simulink model "task11"  (R2023a)
settings: Solver=ode15s  StartTime=0.0  StopTime=10.0  RelTol=1e-3
undefined symbols (not defined in the file or in its folder): DisplayTrajectoryImpedance
settings Model: Creator=LENOVO  LastModifiedBy=LENOVO

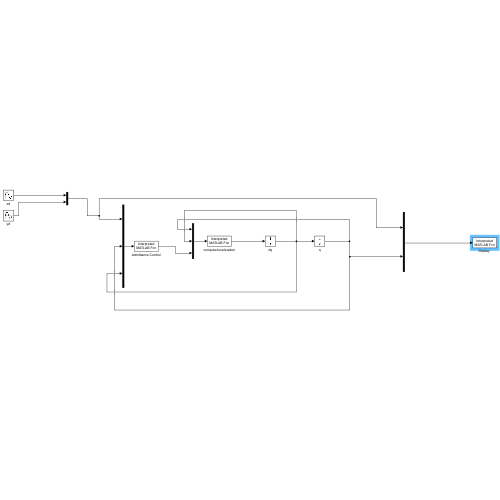
[thumbnail: Simulink's stored preview of the top-level diagram]
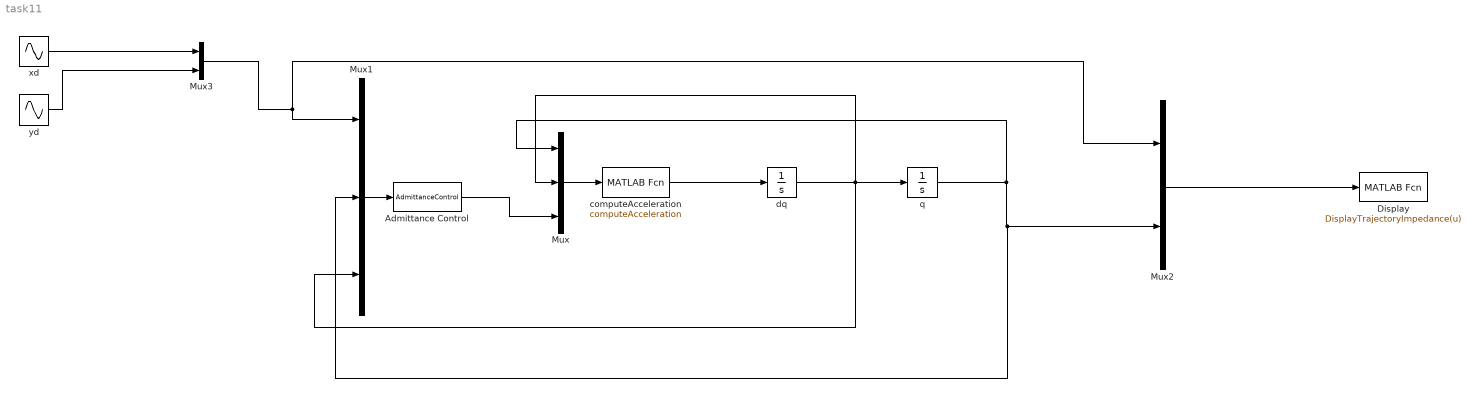
== system task11 ==
  Admittance Control : MATLABFcn  MATLABFcn=AdmittanceControl  OutputDimensions=2
  "Display " : MATLABFcn  MATLABFcn=DisplayTrajectoryImpedance(u)  OutputDimensions=0
  Mux : Mux  Inputs=3
  Mux1 : Mux  Inputs=3
  Mux2 : Mux  Inputs=2
  Mux3 : Mux  Inputs=2
  computeAcceleration : MATLABFcn  MATLABFcn=computeAcceleration  OutputDimensions=2  Output1D=off
  dq : Integrator  InitialCondition=[0; 0]
  q : Integrator  InitialCondition=[pi/2; pi/4]
  xd : Sin  Amplitude=0.1  Bias=0.2  Frequency=0.8*2*pi  Phase=90  SampleTime=0
  yd : Sin  Amplitude=0.3  Bias=0.2  Frequency=0.8*2*pi  SampleTime=0
  wires:
  yd/1 -> Mux3/2
  computeAcceleration/1 -> dq/1
  Mux/1 -> computeAcceleration/1
  dq/1 -> Mux1/3, Mux/2, q/1
  q/1 -> Mux1/2, Mux2/2, Mux/1
  xd/1 -> Mux3/1
  Mux3/1 -> Mux2/1, Mux1/1
  Mux1/1 -> Admittance Control/1
  Admittance Control/1 -> Mux/3
  Mux2/1 -> "Display "/1
